simulink model "ISC_laboratorio_02_01"  (R2019a)
settings: Solver=FixedStepAuto  StartTime=0.0  StopTime=10  FixedStep=1e-2  RelTol=1e-3
undefined symbols (not defined in the file): x0
settings Model: Creator=guilh  LastModifiedBy=guilh
settings DataIOCC: SaveOutput=off  SignalLogging=off  DSMLogging=off  ReturnWorkspaceOutputs=off  TimeSaveName=t

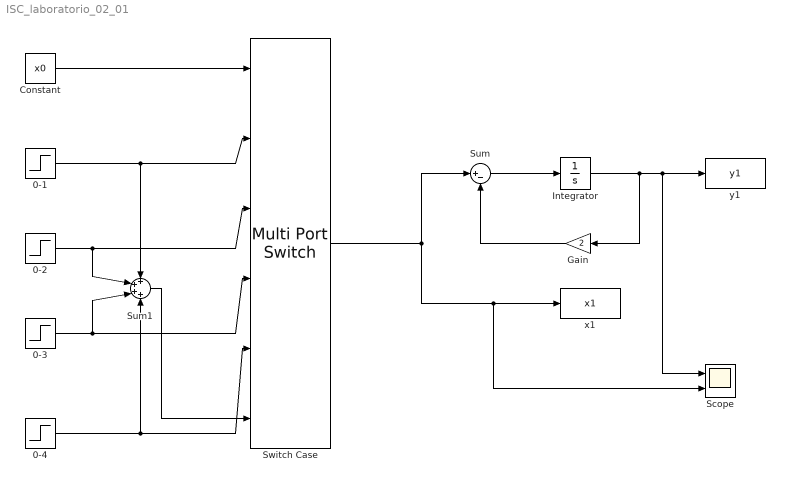
== system ISC_laboratorio_02_01 ==
  0-1 : Step  Time=0  SampleTime=0
  0-2 : Step  Time=0  After=2  SampleTime=0
  0-3 : Step  Time=0  After=3  SampleTime=0
  0-4 : Step  Time=0  After=4  SampleTime=0
  Constant : Constant  Value=x0
  Gain : Gain  Gain=2
  Integrator : Integrator
  Scope : Scope  NumInputPorts=2
  Sum : Sum  Inputs=|+-
  Sum1 : Sum  Inputs=++++
  Switch Case : MultiPortSwitch  Inputs=5
  x1 : ToWorkspace  VariableName=x1  SampleTime=-1
  y1 : ToWorkspace  VariableName=y1  SampleTime=-1
  wires:
  Gain/1 -> Sum/2
  Sum/1 -> Integrator/1
  Switch Case/1 -> Sum/1, Scope/2, x1/1
  0-4/1 -> Switch Case/5, Sum1/4
  0-3/1 -> Switch Case/4, Sum1/3
  0-2/1 -> Sum1/2, Switch Case/3
  0-1/1 -> Sum1/1, Switch Case/2
  Integrator/1 -> Gain/1, Scope/1, y1/1
  Constant/1 -> Switch Case/1
  Sum1/1 -> Switch Case/6
